simulink model "Sim_Ex22"  (R2025a)
settings: Solver=VariableStepAuto  StartTime=0.0  StopTime=Stop_Time  RelTol=1e-3
values from neighbouring files (symbols this model uses):
  L = 1e-3    (= 0.001)    [A_Ex22.m]
  R = 1    [A_Ex22.m]
  Ts = 1/fs    (= 5e-05)    [A_Ex22.m]
  Tsw = 1/fsw    (= 0.0001)    [A_Ex22.m]
  V = Vdc/sqrt(3)*0.7    [A_Ex22.m]
  Vdc = 250    [A_Ex22.m]
  W = 2*pi*500    (= 3141.59265359)    [A_Ex22.m]
undefined symbols (not defined in the file or in its folder): DiscIntNeverNeededParam, Mode
libraries: simulink x2
settings Model: Creator=KYC  LastModifiedBy=New
settings SolverCC: AlgebraicLoopSolver=TrustRegion
settings DataIOCC: ReturnWorkspaceOutputs=off
settings DebuggingCC: UnconnectedInputMsg=warning  UnconnectedOutputMsg=warning  UnconnectedLineMsg=warning  ArithmeticOperatorsInVariantConditions=warning
settings ModelReferenceCC: EnableRefExpFcnMdlSchedulingChecks=on
settings SFSimCC: SimUseLocalCustomCode=off  CustomCodeUndefinedFunction=UseInterfaceOnly
settings RTWCC: RTWUseLocalCustomCode=off  GPUComputeCapability=3.5
settings CodeAppCC: StateflowObjectComments=on

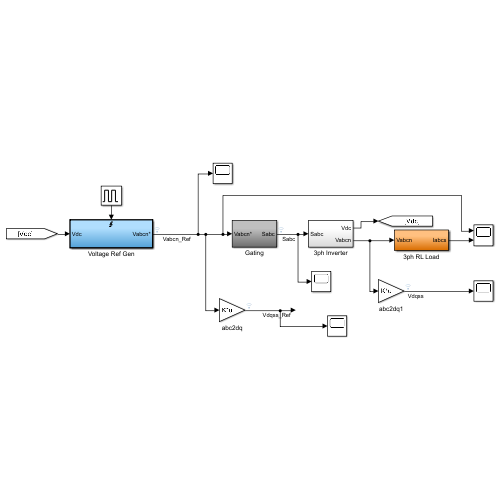
[thumbnail: Simulink's stored preview of the top-level diagram]
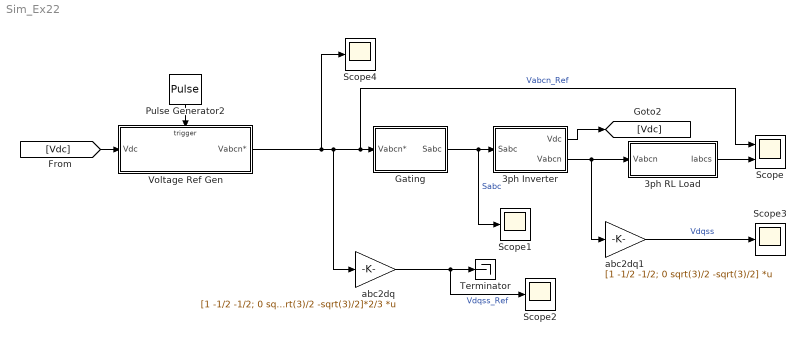
== system Sim_Ex22 ==
  3ph Inverter : Subsystem
  3ph RL Load : Subsystem
  Gating : Subsystem
  Pulse Generator2 : DiscretePulseGenerator  PulseType=Time based  Period=Ts  PulseWidth=50
  Scope : Scope  NumInputPorts=2
      settings: ActiveDisplayYMinimum=-200  ActiveDisplayYMaximum=200
  Scope{1..4} (4 alike) : Scope
      Scope1 settings: ActiveDisplayYMinimum=-0.12499999999999997  ActiveDisplayYMaximum=1.125  DataLoggingVariableName=ScopeData4
      Scope2 settings: ActiveDisplayYMinimum=-126.29537138523064  ActiveDisplayYMaximum=126.29537138523064  DataLoggingVariableName=ScopeData5
      Scope3 settings: ActiveDisplayYMinimum=-312.5  ActiveDisplayYMaximum=312.5  DataLoggingVariableName=ScopeData6
      Scope4 settings: ActiveDisplayYMinimum=-2.34706574074351  ActiveDisplayYMaximum=36.918532179533784  DataLoggingVariableName=ScopeData8
  Terminator : Terminator
  Voltage Ref Gen : Subsystem
  abc2dq : Gain  Gain=[1 -1/2 -1/2; 0 sqrt(3)/2 -sqrt(3)/2]*2/3  Multiplication=Matrix(K*u)
  abc2dq1 : Gain  Gain=[1 -1/2 -1/2; 0 sqrt(3)/2 -sqrt(3)/2]  Multiplication=Matrix(K*u)
  wires:
  Pulse Generator2/1 -> Voltage Ref Gen/Trigger
  Gating/1(Sabc) -> Scope1/1, 3ph Inverter/1(Sabc)  "Sabc"
  3ph Inverter/2(Vabcn) -> abc2dq1/1, 3ph RL Load/1(Vabcn)
  3ph Inverter/1(Vdc) -> [Vdc]
  [Vdc] -> Voltage Ref Gen/1(Vdc)
  3ph RL Load/1(Iabcs) -> Scope/2
  Voltage Ref Gen/1(Vabcn*) -> Scope/1, Gating/1(Vabcn*), abc2dq/1, Scope4/1  "Vabcn_Ref"
  abc2dq/1 -> Scope2/1, Terminator/1  "Vdqss_Ref"
  abc2dq1/1 -> Scope3/1  "Vdqss"

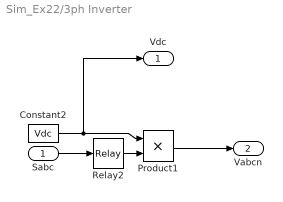
== system Sim_Ex22/3ph Inverter ==
  Sabc : Inport
  Constant2 : Constant  Value=Vdc
  Product1 : Product  RndMeth=Zero
  Relay2 : Relay  OnSwitchValue=0.5  OffSwitchValue=0.5  OnOutputValue=1/2  OffOutputValue=-1/2  OutDataTypeStr=double
  Vdc : Outport
  Vabcn : Outport  Port=2
  wires:
  Constant2/1 -> Vdc/1, Product1/1
  Sabc/1 -> Relay2/1
  Relay2/1 -> Product1/2
  Product1/1 -> Vabcn/1

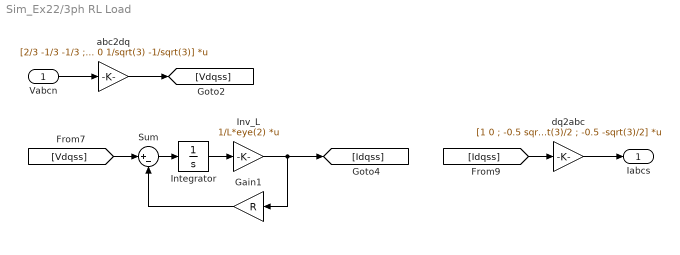
== system Sim_Ex22/3ph RL Load ==
  Vabcn : Inport
  Gain1 : Gain  Gain=R
  Integrator : Integrator
  Inv_L : Gain  Gain=1/L*eye(2)  Multiplication=Matrix(K*u)
  Sum : Sum  Inputs=|+-
  abc2dq : Gain  Gain=[2/3 -1/3 -1/3 ; 0 1/sqrt(3) -1/sqrt(3)]  Multiplication=Matrix(K*u)  SaturateOnIntegerOverflow=on  OutDataTypeStr=Inherit: Same as input  ParamDataTypeStr=Inherit: Same as input
  dq2abc : Gain  Gain=[1 0 ; -0.5 sqrt(3)/2 ; -0.5 -sqrt(3)/2]  Multiplication=Matrix(K*u)
  Iabcs : Outport
  wires:
  abc2dq/1 -> [Vdqss]
  Vabcn/1 -> abc2dq/1
  Gain1/1 -> Sum/2
  Sum/1 -> Integrator/1
  [Vdqss] -> Sum/1
  Integrator/1 -> Inv_L/1
  Inv_L/1 -> [Idqss], Gain1/1
  [Idqss] -> dq2abc/1
  dq2abc/1 -> Iabcs/1

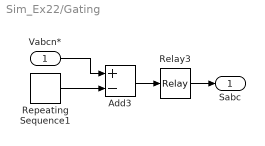
== system Sim_Ex22/Gating ==
  Vabcn* : Inport
  Add3 : Sum  Inputs=+-
  Relay3 : Relay  OnSwitchValue=10*eps  OffSwitchValue=-10*eps  OutDataTypeStr=double
  Repeating Sequence1 : simulink/Sources/Repeating Sequence  rep_seq_t=[0 Tsw/2 Tsw]  rep_seq_y=Vdc*[-0.5 0.5 0-0.5]
  Sabc : Outport
  wires:
  Add3/1 -> Relay3/1
  Vabcn*/1 -> Add3/1
  Relay3/1 -> Sabc/1
  Repeating Sequence1/1 -> Add3/2

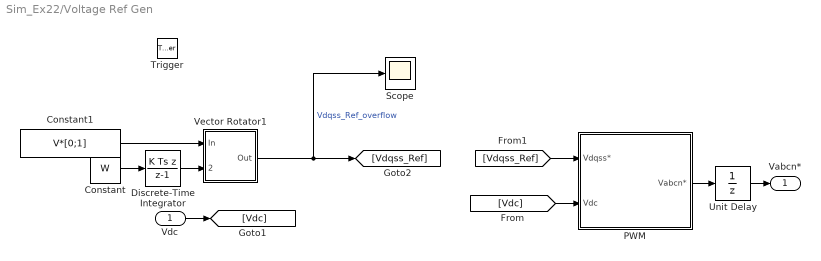
== system Sim_Ex22/Voltage Ref Gen ==
  Vdc : Inport
  Trigger : TriggerPort  VariantControl=Variant  PortDimensions=1
  Constant : Constant  Value=W
  Constant1 : Constant  Value=V*[0;1]
  Discrete-Time Integrator : DiscreteIntegrator  IntegratorMethod=Integration: Backward Euler  SampleTime=-1  ICPrevOutput=DiscIntNeverNeededParam  ICPrevScaledInput=DiscIntNeverNeededParam
  PWM : Subsystem
  Scope : Scope
      settings: ActiveDisplayYMinimum=96.870152215892  ActiveDisplayYMaximum=102.13043617080677  DataLoggingVariableName=ScopeData7
  Unit Delay : UnitDelay  SampleTime=-1  HasFrameUpgradeWarning=on
  Vector Rotator1 : Subsystem
  Vabcn* : Outport  InitialOutput=[0]
  wires:
  Unit Delay/1 -> Vabcn*/1
  Constant/1 -> Discrete-Time Integrator/1
  Discrete-Time Integrator/1 -> Vector Rotator1/2(Theta)
  Constant1/1 -> Vector Rotator1/1(In)
  Vector Rotator1/1(Out) -> Scope/1, [Vdqss_Ref]  "Vdqss_Ref_overflow"
  [Vdqss_Ref] -> PWM/1(Vdqss*)
  PWM/1(Vabcn*) -> Unit Delay/1
  Vdc/1 -> [Vdc]
  [Vdc] -> PWM/2(Vdc)

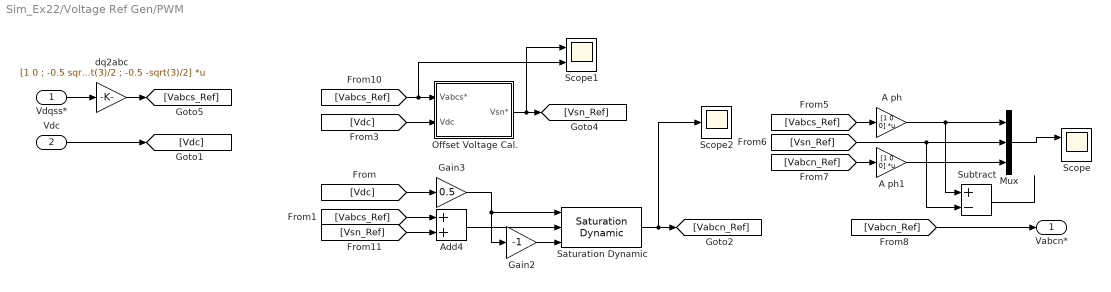
== system Sim_Ex22/Voltage Ref Gen/PWM ==
  Vdqss* : Inport
  Vdc : Inport  Port=2
  A ph : Gain  Gain=[1 0 0]  Multiplication=Matrix(K*u)
  A ph1 : Gain  Gain=[1 0 0]  Multiplication=Matrix(K*u)
  Add4 : Sum
  Gain2 : Gain  Gain=-1
  Gain3 : Gain  Gain=0.5
  Mux : Mux  Inputs=3
  Offset Voltage Cal. : Subsystem
  Saturation Dynamic : simulink/Discontinuities/Saturation Dynamic  OutMin=[]  OutMax=[]  OutDataTypeStr=Inherit: Same as second input  OutDataType=fixdt(1, 16)  OutScaling=2^-10  DoSatur=off
  Scope : Scope  NumInputPorts=2
      settings: ActiveDisplayYMinimum=-112.48728193047992  ActiveDisplayYMaximum=124.97519721471944
  Scope1 : Scope  NumInputPorts=2
      settings: ActiveDisplayYMinimum=-126.29537138523064  ActiveDisplayYMaximum=126.29537138523064  DataLoggingVariableName=ScopeData2
  Scope2 : Scope
      settings: ActiveDisplayYMinimum=101.27314814814815  ActiveDisplayYMaximum=130.20833333333334  DataLoggingVariableName=ScopeData3
  Subtract : Sum  Inputs=+-
  dq2abc : Gain  Gain=[1 0 ; -0.5 sqrt(3)/2 ; -0.5 -sqrt(3)/2]  Multiplication=Matrix(K*u)
  Vabcn* : Outport
  wires:
  Vdqss*/1 -> dq2abc/1
  dq2abc/1 -> [Vabcs_Ref]
  [Vabcs_Ref] -> Add4/1
  [Vsn_Ref] -> Add4/2
  Gain3/1 -> Saturation Dynamic/1, Gain2/1
  Gain2/1 -> Saturation Dynamic/3
  Add4/1 -> Saturation Dynamic/2
  Vdc/1 -> [Vdc]
  [Vdc] -> Gain3/1
  Mux/1 -> Scope/1
  [Vabcs_Ref] -> A ph/1
  A ph/1 -> Subtract/1, Mux/1
  [Vsn_Ref] -> Mux/2, Subtract/2
  A ph1/1 -> Mux/3
  [Vabcn_Ref] -> A ph1/1
  Saturation Dynamic/1 -> Scope2/1, [Vabcn_Ref]
  [Vabcn_Ref] -> Vabcn*/1
  Offset Voltage Cal./1(Vsn*) -> Scope1/1, [Vsn_Ref]
  [Vdc] -> Offset Voltage Cal./2(Vdc)
  [Vabcs_Ref] -> Scope1/2, Offset Voltage Cal./1(Vabcs*)
  Subtract/1 -> ?

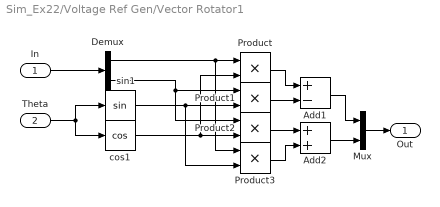
== system Sim_Ex22/Voltage Ref Gen/Vector Rotator1 ==
  In : Inport
  Theta : Inport  Port=2
  Add1 : Sum  Inputs=+-
  Add2 : Sum
  Demux : Demux  Outputs=2
  Mux : Mux  Inputs=[1 1]
  Product{,1..3} (4 alike) : Product  RndMeth=Zero
  cos1 : Trigonometry  Operator=cos
  sin1 : Trigonometry
  Out : Outport
  wires:
  Theta/1 -> cos1/1, sin1/1
  Demux/1 -> Product3/1, Product/1
  Mux/1 -> Out/1
  In/1 -> Demux/1
  Demux/2 -> Product1/1, Product2/1
  cos1/1 -> Product/2, Product2/2
  sin1/1 -> Product1/2, Product3/2
  Product/1 -> Add1/1
  Product1/1 -> Add1/2
  Add1/1 -> Mux/1
  Product2/1 -> Add2/1
  Product3/1 -> Add2/2
  Add2/1 -> Mux/2

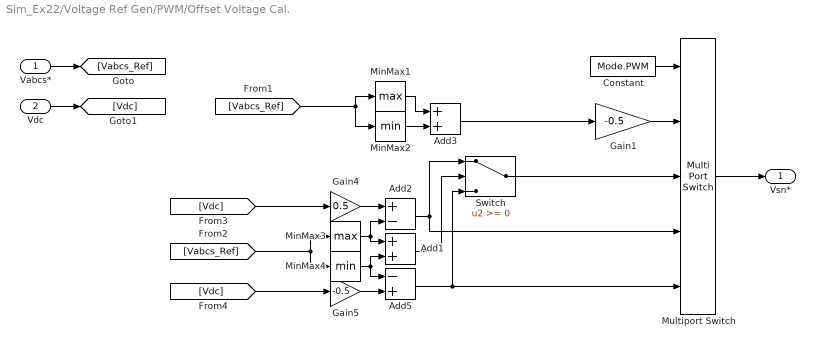
== system Sim_Ex22/Voltage Ref Gen/PWM/Offset Voltage Cal. ==
  Vabcs* : Inport
  Vdc : Inport  Port=2
  Add1 : Sum
  Add2 : Sum  Inputs=+-
  Add3 : Sum
  Add5 : Sum  Inputs=-+
  Constant : Constant  Value=Mode.PWM
  Gain1 : Gain  Gain=-0.5
  Gain4 : Gain  Gain=0.5
  Gain5 : Gain  Gain=-0.5
  MinMax1 : MinMax  Function=max
  MinMax2 : MinMax
  MinMax3 : MinMax  Function=max
  MinMax4 : MinMax
  Multiport Switch : MultiPortSwitch  Inputs=4  SaturateOnIntegerOverflow=off  InputSameDT=off
  Switch : Switch  SaturateOnIntegerOverflow=off  InputSameDT=off
  Vsn* : Outport
  wires:
  Add2/1 -> Multiport Switch/4, Switch/1
  Add3/1 -> Gain1/1
  MinMax2/1 -> Add3/2
  MinMax1/1 -> Add3/1
  Constant/1 -> Multiport Switch/1
  Gain1/1 -> Multiport Switch/2
  MinMax3/1 -> Add2/2, Add1/1
  [Vabcs_Ref] -> MinMax3/1, MinMax4/1
  [Vabcs_Ref] -> MinMax2/1, MinMax1/1
  Multiport Switch/1 -> Vsn*/1
  Add1/1 -> Switch/2
  MinMax4/1 -> Add1/2, Add5/1
  Gain4/1 -> Add2/1
  Switch/1 -> Multiport Switch/3
  [Vdc] -> Gain5/1
  Gain5/1 -> Add5/2
  Add5/1 -> Switch/3, Multiport Switch/5
  [Vdc] -> Gain4/1
  Vabcs*/1 -> [Vabcs_Ref]
  Vdc/1 -> [Vdc]
